simulink model "flowDynamicModel"  (R2022a)
settings: Solver=VariableStepAuto  StartTime=0.0  StopTime=10.0  RelTol=1e-3
settings Model: Creator=a2367980  LastModifiedBy=a2367980

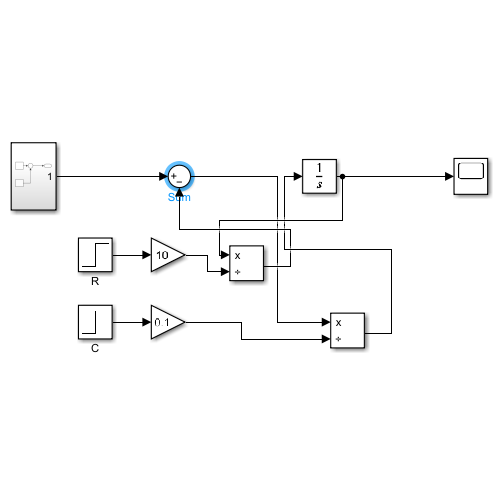
[thumbnail: Simulink's stored preview of the top-level diagram]
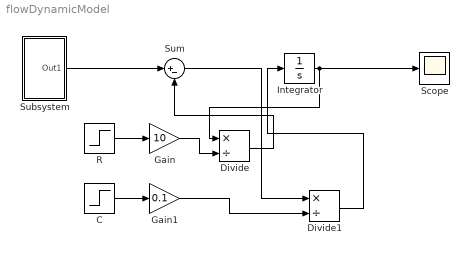
== system flowDynamicModel ==
  C : Step  Time=0  SampleTime=0
  Divide : Product  Inputs=*/
  Divide1 : Product  Inputs=*/
  Gain : Gain  Gain=10
  Gain1 : Gain  Gain=0.1
  Integrator : Integrator
  R : Step  Time=0  SampleTime=0
  Scope : Scope
  Subsystem : Subsystem
  Sum : Sum  Inputs=|+-
  wires:
  Subsystem/1(Out1) -> Sum/1
  R/1 -> Gain/1
  C/1 -> Gain1/1
  Gain/1 -> Divide/2
  Integrator/1 -> Divide/1, Scope/1
  Gain1/1 -> Divide1/2
  Divide/1 -> Sum/2
  Sum/1 -> Divide1/1
  Divide1/1 -> Integrator/1

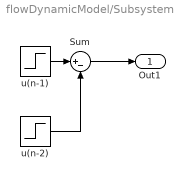
== system flowDynamicModel/Subsystem ==
  Sum : Sum  Inputs=|+-
  u(n-1) : Step  SampleTime=0
  u(n-2) : Step  Time=5  SampleTime=0
  Out1 : Outport
  wires:
  u(n-1)/1 -> Sum/1
  Sum/1 -> Out1/1
  u(n-2)/1 -> Sum/2
